simulink model "Part6PID"  (R2022b)
settings: Solver=VariableStepAuto  StartTime=0.0  StopTime=10.0  RelTol=1e-3
values from neighbouring files (symbols this model uses):
  b = .5    (= 0.5)    [initPart6PID.m]    (also in initRho.m; mobileRobot.m = 0.1; outerLoopInit.m)
  J = .05    (= 0.05)    [initPart6PID.m]    (also in initRho.m; outerLoopInit.m)
  Ke = .5    (= 0.5)    [initPart6PID.m]    (also in initRho.m; outerLoopInit.m)
  Kt = .5    (= 0.5)    [initPart6PID.m]    (also in initRho.m; outerLoopInit.m)
  phi_0 = 0    [initPart6PID.m]
  Ra = 1    [initPart6PID.m]    (also in initRho.m; outerLoopInit.m)
  rhoDot_d = .1    (= 0.1)    [initPart6PID.m]
  x_0 = 0    [initPart6PID.m]
  x_s = [0 0 6 10]    [initPart6PID.m]
  y_0 = 0    [initPart6PID.m]
  y_s = [0 0.25 0 0]    [initPart6PID.m]
libraries: slpidlib x3
settings Model: Creator=ogel0  LastModifiedBy=ogel0

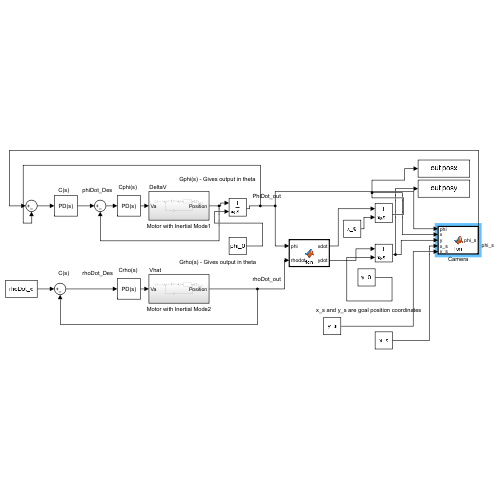
[thumbnail: Simulink's stored preview of the top-level diagram]
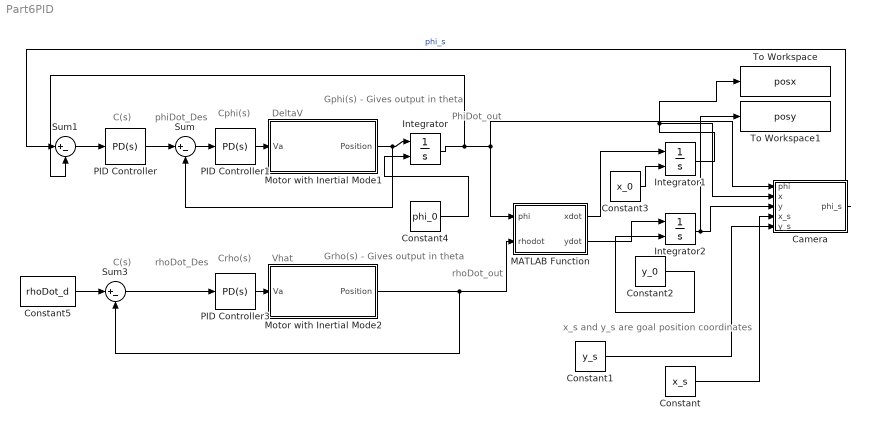
== system Part6PID ==
  note: x_s and y_s are goal position coordinates
  note: DeltaV
  note: C(s)
  note: PhiDot_out
  note: phiDot_Des
  note: Cphi(s)
  note: Gphi(s) - Gives output in theta
  note: Vhat
  note: Grho(s) - Gives output in theta
  note: Crho(s)
  note: rhoDot_out
  note: rhoDot_Des
  note: C(s)
  Camera : MATLAB Function  TreatAsAtomicUnit=on  SystemSampleTime=.2
  Constant : Constant  Value=x_s
  Constant1 : Constant  Value=y_s
  Constant2 : Constant  Value=y_0
  Constant3 : Constant  Value=x_0
  Constant4 : Constant  Value=phi_0
  Constant5 : Constant  Value=rhoDot_d
  Integrator : Integrator  InitialConditionSource=external
  Integrator1 : Integrator  InitialConditionSource=external
  Integrator2 : Integrator  InitialConditionSource=external
  MATLAB Function : MATLAB Function  TreatAsAtomicUnit=on
  Motor with Inertial Mode1 : Subsystem
  Motor with Inertial Mode2 : Subsystem
  PID Controller : slpidlib/PID Controller  Controller=PD  Form=Parallel  TimeDomain=Continuous-time  UseExternalTs=off  SampleTime=-1  IntegratorMethod=Forward Euler  FilterMethod=Forward Euler  ControllerParametersSource=internal  P=55.2518209912998  I=1  UseKiTs=off  D=1.74562338241798  N=5622.73152911984  UseFilter=on  TunerSelectOption=Transfer Function Based (PID Tuner App)  InitialConditionSource=internal  InitialConditionForIntegrator=0  InitialConditionForFilter=0  DifferentiatorICPrevScaledInput=0  ExternalReset=none  TrackingMode=off  Kt=1  LimitOutput=off  SatLimitsSource=internal  UpperSaturationLimit=inf  LowerSaturationLimit=-inf  LinearizeAsGain=on  AntiWindupMode=none  Kb=1  LimitIntegrator=off  UpperIntegratorSaturationLimit=inf  LowerIntegratorSaturationLimit=-inf  POutMin=[]  POutMax=[]  IOutMin=[]  IOutMax=[]  DOutMin=[]  DOutMax=[]  NOutMin=[]  NOutMax=[]  SumOutMin=[]  SumOutMax=[]  SaturationOutMin=[]  SaturationOutMax=[]  PParamMin=[]  PParamMax=[]  IParamMin=[]  IParamMax=[]  DParamMin=[]  DParamMax=[]  NParamMin=[]  NParamMax=[]  KbParamMin=[]  KbParamMax=[]  KtParamMin=[]  KtParamMax=[]  KbOutMin=[]  KbOutMax=[]  KtOutMin=[]  KtOutMax=[]  IntegratorOutMin=[]  IntegratorOutMax=[]  FilterOutMin=[]  FilterOutMax=[]  SumI1OutMin=[]  SumI1OutMax=[]  SumI2OutMin=[]  SumI2OutMax=[]  SumI3OutMin=[]  SumI3OutMax=[]  SumI4OutMin=[]  SumI4OutMax=[]  SumDOutMin=[]  SumDOutMax=[]  DifferentiatorOutMin=[]  DifferentiatorOutMax=[]  FilterDiffOutCoefMin=[]  FilterDiffOutCoefMax=[]  ReciprocalOutMin=[]  ReciprocalOutMax=[]  SumDenOutMin=[]  SumDenOutMax=[]  SumNumOutMin=[]  SumNumOutMax=[]  DivideOutMin=[]  DivideOutMax=[]  UdiffTsProdOutMin=[]  UdiffTsProdOutMax=[]  NTsProdOutMin=[]  NTsProdOutMax=[]  UintegralTsProdOutMin=[]  UintegralTsProdOutMax=[]  UngainTsProdOutMin=[]  UngainTsProdOutMax=[]  ClampingZeroOutDataTypeStr=Inherit: Inherit via back propagation  ClampingZeroOutMin=[]  ClampingZeroOutMax=[]  FilterDenConstantOutDataTypeStr=Inherit: Inherit via back propagation  FilterDenConstantOutMin=[]  FilterDenConstantOutMax=[]  PCopyOutDataTypeStr=Inherit: Inherit via back propagation  PCopyOutMin=[]  PCopyOutMax=[]  NCopyOutDataTypeStr=Inherit: Inherit via back propagation  NCopyOutMin=[]  NCopyOutMax=[]  IntegratorContinuousStateAttributes=''  IntegratorStateMustResolveToSignalObject=off  IntegratorRTWStateStorageClass=Auto  FilterContinuousStateAttributes=''  FilterStateMustResolveToSignalObject=off  FilterRTWStateStorageClass=Auto  ParallelPVariant=InternalParameters  IdealPVariant=Disabled  IVariant=Disabled  DVariant=InternalParameters  IntegratorVariant=Disabled  SatVariant=Disabled  AWVariant=Disabled  PCopyVariant=Disabled  TRVariant=Disabled  FdbkBlocksVariant=Forward  IdealPFdbkVariant=Disabled  SatFdbkVariant=Disabled  DerivativeFilterVariant=ContFilter  NVariant=InternalParameters  NCopyVariant=Disabled  FilterICVariant=InternalICsFilter  IntegratorICVariant=Disabled  ExternalResetVariant=Disabled  TRSumVariant=Passthrough  SumFdbkVariant=Disabled  SumVariant=Sum_PD  TsampFilterVariant=InternalTs  TsampNgainVariant=Passthrough  TsampIntegralVariant=Disabled_SignalSpec  ExternalSaturationOutDataTypeStr=Inherit: Same as second input
  PID Controller1 : slpidlib/PID Controller  Controller=PD  Form=Parallel  TimeDomain=Continuous-time  UseExternalTs=off  SampleTime=-1  IntegratorMethod=Forward Euler  FilterMethod=Forward Euler  ControllerParametersSource=internal  P=44.9539024669916  I=1  UseKiTs=off  D=2.54579413878844  N=3053.09155413539  UseFilter=on  TunerSelectOption=Transfer Function Based (PID Tuner App)  InitialConditionSource=internal  InitialConditionForIntegrator=0  InitialConditionForFilter=0  DifferentiatorICPrevScaledInput=0  ExternalReset=none  TrackingMode=off  Kt=1  LimitOutput=off  SatLimitsSource=internal  UpperSaturationLimit=inf  LowerSaturationLimit=-inf  LinearizeAsGain=on  AntiWindupMode=none  Kb=1  LimitIntegrator=off  UpperIntegratorSaturationLimit=inf  LowerIntegratorSaturationLimit=-inf  POutMin=[]  POutMax=[]  IOutMin=[]  IOutMax=[]  DOutMin=[]  DOutMax=[]  NOutMin=[]  NOutMax=[]  SumOutMin=[]  SumOutMax=[]  SaturationOutMin=[]  SaturationOutMax=[]  PParamMin=[]  PParamMax=[]  IParamMin=[]  IParamMax=[]  DParamMin=[]  DParamMax=[]  NParamMin=[]  NParamMax=[]  KbParamMin=[]  KbParamMax=[]  KtParamMin=[]  KtParamMax=[]  KbOutMin=[]  KbOutMax=[]  KtOutMin=[]  KtOutMax=[]  IntegratorOutMin=[]  IntegratorOutMax=[]  FilterOutMin=[]  FilterOutMax=[]  SumI1OutMin=[]  SumI1OutMax=[]  SumI2OutMin=[]  SumI2OutMax=[]  SumI3OutMin=[]  SumI3OutMax=[]  SumI4OutMin=[]  SumI4OutMax=[]  SumDOutMin=[]  SumDOutMax=[]  DifferentiatorOutMin=[]  DifferentiatorOutMax=[]  FilterDiffOutCoefMin=[]  FilterDiffOutCoefMax=[]  ReciprocalOutMin=[]  ReciprocalOutMax=[]  SumDenOutMin=[]  SumDenOutMax=[]  SumNumOutMin=[]  SumNumOutMax=[]  DivideOutMin=[]  DivideOutMax=[]  UdiffTsProdOutMin=[]  UdiffTsProdOutMax=[]  NTsProdOutMin=[]  NTsProdOutMax=[]  UintegralTsProdOutMin=[]  UintegralTsProdOutMax=[]  UngainTsProdOutMin=[]  UngainTsProdOutMax=[]  ClampingZeroOutDataTypeStr=Inherit: Inherit via back propagation  ClampingZeroOutMin=[]  ClampingZeroOutMax=[]  FilterDenConstantOutDataTypeStr=Inherit: Inherit via back propagation  FilterDenConstantOutMin=[]  FilterDenConstantOutMax=[]  PCopyOutDataTypeStr=Inherit: Inherit via back propagation  PCopyOutMin=[]  PCopyOutMax=[]  NCopyOutDataTypeStr=Inherit: Inherit via back propagation  NCopyOutMin=[]  NCopyOutMax=[]  IntegratorContinuousStateAttributes=''  IntegratorStateMustResolveToSignalObject=off  IntegratorRTWStateStorageClass=Auto  FilterContinuousStateAttributes=''  FilterStateMustResolveToSignalObject=off  FilterRTWStateStorageClass=Auto  ParallelPVariant=InternalParameters  IdealPVariant=Disabled  IVariant=Disabled  DVariant=InternalParameters  IntegratorVariant=Disabled  SatVariant=Disabled  AWVariant=Disabled  PCopyVariant=Disabled  TRVariant=Disabled  FdbkBlocksVariant=Forward  IdealPFdbkVariant=Disabled  SatFdbkVariant=Disabled  DerivativeFilterVariant=ContFilter  NVariant=InternalParameters  NCopyVariant=Disabled  FilterICVariant=InternalICsFilter  IntegratorICVariant=Disabled  ExternalResetVariant=Disabled  TRSumVariant=Passthrough  SumFdbkVariant=Disabled  SumVariant=Sum_PD  TsampFilterVariant=InternalTs  TsampNgainVariant=Passthrough  TsampIntegralVariant=Disabled_SignalSpec  ExternalSaturationOutDataTypeStr=Inherit: Same as second input
  PID Controller3 : slpidlib/PID Controller  Controller=PD  Form=Parallel  TimeDomain=Continuous-time  UseExternalTs=off  SampleTime=-1  IntegratorMethod=Forward Euler  FilterMethod=Forward Euler  ControllerParametersSource=internal  P=44.9539024669916  I=1  UseKiTs=off  D=2.54579413878844  N=3053.09155413539  UseFilter=on  TunerSelectOption=Transfer Function Based (PID Tuner App)  InitialConditionSource=internal  InitialConditionForIntegrator=0  InitialConditionForFilter=0  DifferentiatorICPrevScaledInput=0  ExternalReset=none  TrackingMode=off  Kt=1  LimitOutput=off  SatLimitsSource=internal  UpperSaturationLimit=inf  LowerSaturationLimit=-inf  LinearizeAsGain=on  AntiWindupMode=none  Kb=1  LimitIntegrator=off  UpperIntegratorSaturationLimit=inf  LowerIntegratorSaturationLimit=-inf  POutMin=[]  POutMax=[]  IOutMin=[]  IOutMax=[]  DOutMin=[]  DOutMax=[]  NOutMin=[]  NOutMax=[]  SumOutMin=[]  SumOutMax=[]  SaturationOutMin=[]  SaturationOutMax=[]  PParamMin=[]  PParamMax=[]  IParamMin=[]  IParamMax=[]  DParamMin=[]  DParamMax=[]  NParamMin=[]  NParamMax=[]  KbParamMin=[]  KbParamMax=[]  KtParamMin=[]  KtParamMax=[]  KbOutMin=[]  KbOutMax=[]  KtOutMin=[]  KtOutMax=[]  IntegratorOutMin=[]  IntegratorOutMax=[]  FilterOutMin=[]  FilterOutMax=[]  SumI1OutMin=[]  SumI1OutMax=[]  SumI2OutMin=[]  SumI2OutMax=[]  SumI3OutMin=[]  SumI3OutMax=[]  SumI4OutMin=[]  SumI4OutMax=[]  SumDOutMin=[]  SumDOutMax=[]  DifferentiatorOutMin=[]  DifferentiatorOutMax=[]  FilterDiffOutCoefMin=[]  FilterDiffOutCoefMax=[]  ReciprocalOutMin=[]  ReciprocalOutMax=[]  SumDenOutMin=[]  SumDenOutMax=[]  SumNumOutMin=[]  SumNumOutMax=[]  DivideOutMin=[]  DivideOutMax=[]  UdiffTsProdOutMin=[]  UdiffTsProdOutMax=[]  NTsProdOutMin=[]  NTsProdOutMax=[]  UintegralTsProdOutMin=[]  UintegralTsProdOutMax=[]  UngainTsProdOutMin=[]  UngainTsProdOutMax=[]  ClampingZeroOutDataTypeStr=Inherit: Inherit via back propagation  ClampingZeroOutMin=[]  ClampingZeroOutMax=[]  FilterDenConstantOutDataTypeStr=Inherit: Inherit via back propagation  FilterDenConstantOutMin=[]  FilterDenConstantOutMax=[]  PCopyOutDataTypeStr=Inherit: Inherit via back propagation  PCopyOutMin=[]  PCopyOutMax=[]  NCopyOutDataTypeStr=Inherit: Inherit via back propagation  NCopyOutMin=[]  NCopyOutMax=[]  IntegratorContinuousStateAttributes=''  IntegratorStateMustResolveToSignalObject=off  IntegratorRTWStateStorageClass=Auto  FilterContinuousStateAttributes=''  FilterStateMustResolveToSignalObject=off  FilterRTWStateStorageClass=Auto  ParallelPVariant=InternalParameters  IdealPVariant=Disabled  IVariant=Disabled  DVariant=InternalParameters  IntegratorVariant=Disabled  SatVariant=Disabled  AWVariant=Disabled  PCopyVariant=Disabled  TRVariant=Disabled  FdbkBlocksVariant=Forward  IdealPFdbkVariant=Disabled  SatFdbkVariant=Disabled  DerivativeFilterVariant=ContFilter  NVariant=InternalParameters  NCopyVariant=Disabled  FilterICVariant=InternalICsFilter  IntegratorICVariant=Disabled  ExternalResetVariant=Disabled  TRSumVariant=Passthrough  SumFdbkVariant=Disabled  SumVariant=Sum_PD  TsampFilterVariant=InternalTs  TsampNgainVariant=Passthrough  TsampIntegralVariant=Disabled_SignalSpec  ExternalSaturationOutDataTypeStr=Inherit: Same as second input
  Sum : Sum  Inputs=|+-
  Sum1 : Sum  Inputs=|+-
  Sum3 : Sum  Inputs=|+-
  To Workspace : ToWorkspace  VariableName=posx  SaveFormat=Timeseries  SampleTime=-1
  To Workspace1 : ToWorkspace  VariableName=posy  SaveFormat=Timeseries  SampleTime=-1
  wires:
  PID Controller/1 -> Sum/1
  Motor with Inertial Mode1/1(Position) -> Sum/2, Integrator/1
  Sum1/1 -> PID Controller/1
  Integrator/1 -> MATLAB Function/1(phi), Camera/1(phi), Sum1/2
  PID Controller1/1 -> Motor with Inertial Mode1/1(Va)
  Sum/1 -> PID Controller1/1
  Sum3/1 -> PID Controller3/1
  PID Controller3/1 -> Motor with Inertial Mode2/1(Va)
  Motor with Inertial Mode2/1(Position) -> MATLAB Function/2(rhodot), Sum3/2
  Constant5/1 -> Sum3/1
  Integrator2/1 -> To Workspace1/1, Camera/3(y)
  Integrator1/1 -> To Workspace/1, Camera/2(x)
  Camera/1(phi_s) -> Sum1/1  "phi_s"
  MATLAB Function/2(ydot) -> Integrator2/1
  MATLAB Function/1(xdot) -> Integrator1/1
  Constant/1 -> Camera/4(x_s)
  Constant1/1 -> Camera/5(y_s)
  Constant3/1 -> Integrator1/2
  Constant2/1 -> Integrator2/2
  Constant4/1 -> Integrator/2

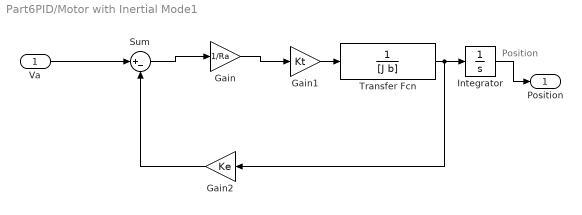
== system Part6PID/Motor with Inertial Mode1 ==
  note: Position
  Va : Inport
  Gain : Gain  Gain=1/Ra
  Gain1 : Gain  Gain=Kt
  Gain2 : Gain  Gain=Ke
  Integrator : Integrator
  Sum : Sum  Inputs=|+-
  Transfer Fcn : TransferFcn  Denominator=[J b]
  Position : Outport
  wires:
  Gain/1 -> Gain1/1
  Transfer Fcn/1 -> Gain2/1, Integrator/1
  Va/1 -> Sum/1
  Sum/1 -> Gain/1
  Gain1/1 -> Transfer Fcn/1
  Gain2/1 -> Sum/2
  Integrator/1 -> Position/1

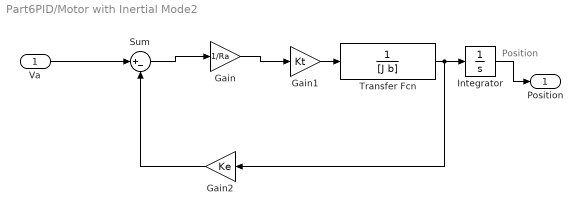
== system Part6PID/Motor with Inertial Mode2 ==
  note: Position
  Va : Inport
  Gain : Gain  Gain=1/Ra
  Gain1 : Gain  Gain=Kt
  Gain2 : Gain  Gain=Ke
  Integrator : Integrator
  Sum : Sum  Inputs=|+-
  Transfer Fcn : TransferFcn  Denominator=[J b]
  Position : Outport
  wires:
  Gain/1 -> Gain1/1
  Transfer Fcn/1 -> Gain2/1, Integrator/1
  Va/1 -> Sum/1
  Sum/1 -> Gain/1
  Gain1/1 -> Transfer Fcn/1
  Gain2/1 -> Sum/2
  Integrator/1 -> Position/1

== matlab function Part6PID/MATLAB Function ==
  data: phi input; xdot output; rhodot input; ydot output
function [xdot,ydot]= fcn(phi,rhodot)

xdot=rhodot*cos(phi*pi/180);
ydot=rhodot*sin(phi*pi/180);

== matlab function Part6PID/Camera ==
  data: phi input; phi_s output; x input; y input; x_s input; y_s input
function phi_s = fcn(phi,x,y,x_s,y_s)
%#codegen
%
% Simulation of Camera with line detection
% phi - angle of robot in degrees
% x - x position of robot in feet
% y - y position of robot in feet
% x_s - vector of x coordinates for line to be detected (in feet)
% y_s - vector of y coordinates for line to be detected (in feet)
%
%

% change show_image to 1 to see camera image during simulation
show_image=1;
%
% number of horizontal and vertical pixels
%
h_pix = 740;
v_pix = 480;
%
% pixel_check is the row of the image to check for the line (origin of
% camera image is upper right
% 
pixel_check = v_pix*4/5;
%
% meters to feet conversion
%
mtof = 3.28;
% f is focal length 
%
f = .0036; %m
f = mtof*f; % convert to feet
%
% sensor image area
%
image_w = .00376; % m
image_h = .00274; % m
image_w = image_w*mtof; % convert to feet
image_h = image_h*mtof; % convert to feet
%
% h is height of the camera 
%
h = 0.1; % m
h = h*mtof; % convert to feet
%
% angle of view is from center to edge of camrea in radians
%
angle_of_view=53.5; % degrees

%
% interpolate between line points
%
x_s = interp1q((1:length(x_s))',x_s,(1:.01:length(x_s))');
y_s = interp1q((1:length(y_s))',y_s,(1:.01:length(y_s))');
%
% translate points to camera origin
% 
tape=[x_s,y_s]';
% figure
% plot(tape(1,:),tape(2,:),'*')
% axis([-5 5 -5 5])

tape = tape - [x;y]*ones(1,size(tape,2));
% figure
% plot(tape(1,:),tape(2,:),'*')
% axis([-5 5 -5 5])
%
% find points that are in the angle of view
%
angle = (180/pi)*acos(([cos(phi*pi/180) sin(phi*pi/180)]*tape)./sqrt(sum(tape.^2)));
index=find(angle<angle_of_view/2 & angle>-angle_of_view/2);
if isempty(index)
    disp('Tape not visible to the robot')
    phi_s = 0;
    return
end;
tape=tape(:,index);
% figure
% plot(tape(1,:),tape(2,:),'*')
% hold on
% fill(v_c(1,:),v_c(2,:),'y')
% title('visible points')
% axis([-5 5 -5 5])
%
% rotate points so straight ahead is along x axis
%
tapenorm=[cos(phi*pi/180) sin(phi*pi/180);-sin(phi*pi/180) cos(phi*pi/180)]*tape;
%
% map onto film coordinates
%
image = [(f./tapenorm(1,:)).*(-tapenorm(2,:));
    (f./tapenorm(1,:)).*(-h*ones(1,size(tapenorm,2)))];
% figure
% plot(image(1,:),image(2,:),'*')
% axis([-image_w/2 image_w/2 -image_h/2 image_h/2])

%
% map onto pixel coordinates
%
pixel = [0; v_pix]*ones(1,size(image,2)) + diag([h_pix/image_w -v_pix/image_h])*image+[h_pix/2; -v_pix/2]*ones(1,size(image,2));
if (show_image)
 figure(1)
 plot(pixel(1,:),pixel(2,:),'*')
 set(gca, 'YDir','reverse')
 hold on
 plot([0 h_pix],[pixel_check pixel_check],'r-')
 axis([0 h_pix 0 v_pix])
 hold off
 title('Robot camera view set show_image=0 to turn off and speed up simulation','interpreter','none')
end;


%
% find point on horizontal line at pixel number pixel_check
%
checkpoints= find(pixel(2,:)>=pixel_check);
if ~isempty(checkpoints)
    [m,index]=min(pixel(2,checkpoints));  
    if abs(pixel(2,index)-pixel_check)>10,
        disp(['no point visible near row ',int2str(pixel_check)])
        phi_s = 0;
        return
    end;
else
    disp(['no point visible near row ',int2str(pixel_check)])
    phi_s = 0;
    return
end;


phi_s = -(pixel(1,index)-h_pix/2)*angle_of_view/h_pix;
